simulink model "big2"  (R2023b)
settings: Solver=VariableStepAuto  StartTime=0.0  StopTime=500  RelTol=1e-3
libraries: simulink x2, aerolibasang x2, simulink_extras x2, aerolibanim x1
(part 3 of 3)

== matlab function big2/Subsystem/Subsystem3/MATLAB Function4 ==
  data: alpha input; DNDR output; beta input
% function DNDR = ddo_lookup(alpha, beta)
%     % Initialize output
%     DNDR = 0; % Ensure DLDN is scalar and fixed size
% 
%     % Declare persistent variables to hold constant data
%     persistent alpha_values beta_values data num_alpha num_beta
% 
%     if isempty(alpha_values)
%         % Initialize alpha and beta values in the table
%         alpha_values = [-10, -5, 0, 5, 10, 15, 20, 25, 30, 35, 40, 45];
%         beta_values  = [-30, -20, -10, 0, 10, 20, 30];
% 
%         num_alpha = length(alpha_values);
%         num_beta = length(beta_values);
% 
%         % Data matrix corresponding to beta (rows) and alpha (columns)
%          data = [
%         -.018, -.052, -.052, -.052, -.054, -.049, -.059, -.051, -.030, -.037, -.026, -.013; % Row for beta = -30
%         -.028, -.051, -.043, -.046, -.045, -.049, -.057, -.052, -.030, -.033, -.030, -.008; % Row for beta = -20°
%         -.037, -.041, -.038, -.040, -.040, -.038, -.037, -.030, -.027, -.024, -.019, -.013; % Row for beta = -10°
%         -.048, -.045, -.045, -.045, -.044, -.045, -.047, -.048, -.049, -.045, -.033, -.016; % Row for beta = 0°
%         -.043, -.044, -.041, -.041, -.040, -.038, -.034, -.035, -.035, -.029, -.022, -.009; % Row for beta = 10°
%         -.052, -.034, -.036, -.036, -.035, -.028, -.024, -.023, -.020, -.016, -.010, -.014; % Row for beta = 20°
%         -.062, -.034, -.027, -.028, -.027, -.027, -.023, -.023, -.019, -.009, -.025, -.010; % Row for beta = 30°
%     ];
%     end
% 
%     % Ensure alpha is within the range; if not, use the closest value
%     alpha_index = int32(1);
%     min_alpha_diff = abs(alpha - alpha_values(1));
%     for i = int32(2):int32(num_alpha)
%         current_diff = abs(alpha - alpha_values(i));
%         if current_diff < min_alpha_diff
%             min_alpha_diff = current_diff;
%             alpha_index = i;
%         end
%     end
% 
%     % Ensure beta is within the range; if not, use the closest value
%     beta_index = int32(1);
%     min_beta_diff = abs(beta - beta_values(1));
%     for i = int32(2):int32(num_beta)
%         current_diff = abs(beta - beta_values(i));
%         if current_diff < min_beta_diff
%             min_beta_diff = current_diff;
%             beta_index = i;
%         end
%     end
% 
%     % Retrieve the corresponding value from the data table
%     DNDR = data(beta_index, alpha_index);
% end
% 
function DNDR = ddo_lookup(alpha, beta)
    % Initialize output
    DNDR = 0; % Ensure DNDR is scalar and fixed size

    % Declare persistent variables to hold constant data
    persistent alpha_values beta_values data num_alpha num_beta

    if isempty(alpha_values)
        % Initialize alpha and beta values in the table
        alpha_values = [-10, -5, 0, 5, 10, 15, 20, 25, 30, 35, 40, 45];
        beta_values  = [-30, -20, -10, 0, 10, 20, 30];

        num_alpha = length(alpha_values);
        num_beta = length(beta_values);

        % Data matrix corresponding to beta (rows) and alpha (columns)
        data = [
            -0.018, -0.052, -0.052, -0.052, -0.054, -0.049, -0.059, -0.051, -0.030, -0.037, -0.026, -0.013; % Beta = -30°
            -0.028, -0.051, -0.043, -0.046, -0.045, -0.049, -0.057, -0.052, -0.030, -0.033, -0.030, -0.008; % Beta = -20°
            -0.037, -0.041, -0.038, -0.040, -0.040, -0.038, -0.037, -0.030, -0.027, -0.024, -0.019, -0.013; % Beta = -10°
            -0.048, -0.045, -0.045, -0.045, -0.044, -0.045, -0.047, -0.048, -0.049, -0.045, -0.033, -0.016; % Beta = 0°
            -0.043, -0.044, -0.041, -0.041, -0.040, -0.038, -0.034, -0.035, -0.035, -0.029, -0.022, -0.009; % Beta = 10°
            -0.052, -0.034, -0.036, -0.036, -0.035, -0.028, -0.024, -0.023, -0.020, -0.016, -0.010, -0.014; % Beta = 20°
            -0.062, -0.034, -0.027, -0.028, -0.027, -0.027, -0.023, -0.023, -0.019, -0.009, -0.025, -0.010; % Beta = 30°
        ];
    end

    % Handle out-of-range alpha values
    if alpha <= alpha_values(1)
        alpha_lower = alpha_values(1);
        alpha_upper = alpha_values(1);
        alpha_idx_lower = int32(1);
        alpha_idx_upper = int32(1);
    elseif alpha >= alpha_values(num_alpha)
        alpha_lower = alpha_values(num_alpha);
        alpha_upper = alpha_values(num_alpha);
        alpha_idx_lower = int32(num_alpha);
        alpha_idx_upper = int32(num_alpha);
    else
        % Find indices for alpha
        alpha_idx_lower = int32(1);
        alpha_idx_upper = int32(1);
        for i = int32(1):(num_alpha - 1)
            if alpha_values(i) <= alpha && alpha < alpha_values(i+1)
                alpha_idx_lower = i;
                alpha_idx_upper = i + 1;
                break;
            end
        end
        alpha_lower = alpha_values(alpha_idx_lower);
        alpha_upper = alpha_values(alpha_idx_upper);
    end

    % Handle out-of-range beta values
    if beta <= beta_values(1)
        beta_lower = beta_values(1);
        beta_upper = beta_values(1);
        beta_idx_lower = int32(1);
        beta_idx_upper = int32(1);
    elseif beta >= beta_values(num_beta)
        beta_lower = beta_values(num_beta);
        beta_upper = beta_values(num_beta);
        beta_idx_lower = int32(num_beta);
        beta_idx_upper = int32(num_beta);
    else
        % Find indices for beta
        beta_idx_lower = int32(1);
        beta_idx_upper = int32(1);
        for i = int32(1):(num_beta - 1)
            if beta_values(i) <= beta && beta < beta_values(i+1)
                beta_idx_lower = i;
                beta_idx_upper = i + 1;
                break;
            end
        end
        beta_lower = beta_values(beta_idx_lower);
        beta_upper = beta_values(beta_idx_upper);
    end

    % Get the four surrounding data points for bilinear interpolation
    Q11 = data(beta_idx_lower, alpha_idx_lower);
    Q12 = data(beta_idx_lower, alpha_idx_upper);
    Q21 = data(beta_idx_upper, alpha_idx_lower);
    Q22 = data(beta_idx_upper, alpha_idx_upper);

    % Perform bilinear interpolation
    if (alpha_upper - alpha_lower) == 0 && (beta_upper - beta_lower) == 0
        % Point lies exactly on a data point
        DNDR = data(beta_idx_lower, alpha_idx_lower);
    elseif (alpha_upper - alpha_lower) == 0
        % Interpolate in beta direction only
        DNDR = Q11 + ((beta - beta_lower) / (beta_upper - beta_lower)) * (Q21 - Q11);
    elseif (beta_upper - beta_lower) == 0
        % Interpolate in alpha direction only
        DNDR = Q11 + ((alpha - alpha_lower) / (alpha_upper - alpha_lower)) * (Q12 - Q11);
    else
        % Full bilinear interpolation
        DNDR = (1 / ((alpha_upper - alpha_lower) * (beta_upper - beta_lower))) * ...
               (Q11 * (alpha_upper - alpha) * (beta_upper - beta) + ...
                Q21 * (alpha - alpha_lower) * (beta_upper - beta) + ...
                Q12 * (alpha_upper - alpha) * (beta - beta_lower) + ...
                Q22 * (alpha - alpha_lower) * (beta - beta_lower));
    end
end

== matlab function big2/Subsystem/Subsystem1/MATLAB Function2 ==
  data: alpha input; c_m output; el input
function c_m = compute_cm_fixed(alpha, el)
    % Embedded data
    data_CM_updated_data_full = [
        0.205, 0.168, 0.186, 0.196, 0.213, 0.251, 0.245, 0.238, 0.252, 0.231, 0.198, 0.192;
        0.081, 0.077, 0.107, 0.110, 0.110, 0.141, 0.127, 0.119, 0.133, 0.108, 0.081, 0.093;
        -0.046, -0.020, -0.009, -0.005, -0.006, 0.010, 0.006, -0.001, 0.014, 0.000, -0.013, 0.032;
        -0.174, -0.145, -0.121, -0.127, -0.129, -0.102, -0.097, -0.113, -0.087, -0.084, -0.069, -0.006;
        -0.259, -0.202, -0.184, -0.193, -0.199, -0.150, -0.160, -0.167, -0.104, -0.076, -0.041, -0.005
    ];

    % Map Alpha and EL into indices and interpolate
    scaled_alpha = 0.2 * alpha;
    k = floor(scaled_alpha);
    k = max(-2, min(k, 8)); % Constrain within bounds
    da = scaled_alpha - k;
    l = k + sign(1.1 * da);
    l = max(-1, min(l, 8)); % Constrain within bounds

    % Adjust indices for MATLAB (1-based indexing)
    k_index = k + 3;
    l_index = l + 3;

    scaled_el = el / 12.5;
    m = floor(scaled_el);
    m = max(-2, min(m, 2)); % Constrain within bounds
    de = scaled_el - m;
    n = m + sign(1.1 * de);
    n = max(-2, min(n, 2)); % Constrain within bounds

    % Adjust indices for MATLAB (1-based indexing)
    m_index = m + 3;
    n_index = n + 3;

    % Interpolate values
    t = data_CM_updated_data_full(m_index, k_index);
    u = data_CM_updated_data_full(n_index, k_index);
    v = t + abs(da) * (data_CM_updated_data_full(m_index, l_index) - t);
    w = u + abs(da) * (data_CM_updated_data_full(n_index, l_index) - u);

    % Final interpolation
    c_m = v + (w - v) * abs(de);
end

== matlab function big2/Subsystem/Subsystem1/MATLAB Function3 ==
  data: alpha input; c_l output; beta input
function c_l = compute_cl_fixed(alpha, beta)
    % Embedded data
    data_CL_updated_data_full = [
        -0.001, -0.004, -0.008, -0.012, -0.016, -0.019, -0.020, -0.020, -0.015, -0.008, -0.013, -0.015;
        -0.003, -0.009, -0.017, -0.024, -0.030, -0.034, -0.040, -0.037, -0.016, -0.002, -0.010, -0.019;
        -0.001, -0.010, -0.020, -0.030, -0.039, -0.044, -0.050, -0.049, -0.023, -0.006, -0.014, -0.027;
        0.000, -0.010, -0.022, -0.034, -0.047, -0.046, -0.059, -0.061, -0.033, -0.036, -0.035, -0.035;
        0.007, -0.010, -0.023, -0.034, -0.049, -0.046, -0.068, -0.071, -0.060, -0.058, -0.062, -0.059;
        0.009, -0.011, -0.023, -0.037, -0.050, -0.047, -0.074, -0.079, -0.091, -0.076, -0.077, -0.076
    ];

    % Scale and map alpha into indices
    scaled_alpha = 0.2 * alpha;
    k = floor(scaled_alpha);                  % Find lower index
    k = max(-2, min(k, 8));                   % Constrain within bounds
    da = scaled_alpha - k;                    % Fractional part for interpolation
    l = k + sign(1.1 * da);                   % Find upper index
    l = max(-2, min(l, 8));                   % Constrain within bounds

    % Adjust indices for MATLAB (1-based indexing)
    k_index = k + 3;                          % Shift index for 1-based indexing
    l_index = l + 3;                          % Shift index for 1-based indexing

    % Scale and map beta into indices
    scaled_beta = 0.2 * abs(beta);
    m = floor(scaled_beta);                   % Find lower index
    m = max(0, min(m, 5));                    % Constrain within bounds
    db = scaled_beta - m;                     % Fractional part for interpolation
    n = m + sign(1.1 * db);                   % Find upper index
    n = max(0, min(n, 5));                    % Constrain within bounds

    % Adjust indices for MATLAB (1-based indexing)
    m_index = m + 1;                          % Shift index for 1-based indexing
    n_index = n + 1;                          % Shift index for 1-based indexing

    % Interpolation in the alpha dimension
    t = data_CL_updated_data_full(m_index, k_index); % Lower beta, lower alpha
    u = data_CL_updated_data_full(n_index, k_index); % Upper beta, lower alpha
    v = t + abs(da) * (data_CL_updated_data_full(m_index, l_index) - t); % Lower beta, interpolated alpha
    w = u + abs(da) * (data_CL_updated_data_full(n_index, l_index) - u); % Upper beta, interpolated alpha

    % Interpolation in the beta dimension
    c_l = v + (w - v) * abs(db);              % Final interpolated value
end

== matlab function big2/Subsystem/Subsystem1/MATLAB Function4 ==
  data: alpha input; c_n output; beta input
function c_n = compute_cn_fixed(alpha, beta)
    % Embedded data
    data_CN_updated_data_full = [
        0.018, 0.019, 0.018, 0.019, 0.019, 0.018, 0.013, 0.007, 0.004, -0.014, -0.017, -0.033;
        0.038, 0.042, 0.042, 0.042, 0.043, 0.039, 0.030, 0.017, 0.004, -0.035, -0.047, -0.057;
        0.056, 0.057, 0.059, 0.058, 0.058, 0.053, 0.032, 0.012, 0.002, -0.046, -0.071, -0.073;
        0.064, 0.077, 0.076, 0.074, 0.073, 0.057, 0.029, 0.007, 0.012, -0.034, -0.065, -0.041;
        0.074, 0.086, 0.093, 0.089, 0.080, 0.062, 0.049, 0.022, 0.028, -0.012, -0.002, -0.013;
        0.079, 0.090, 0.106, 0.106, 0.096, 0.080, 0.068, 0.030, 0.064, 0.015, 0.011, -0.001
    ];

    % Scale and map alpha into indices
    scaled_alpha = 0.2 * alpha;
    k = floor(scaled_alpha);                  % Find lower index
    k = max(-2, min(k, 8));                   % Constrain within bounds
    da = scaled_alpha - k;                    % Fractional part for interpolation
    l = k + sign(1.1 * da);                   % Find upper index
    l = max(-2, min(l, 8));                   % Constrain within bounds

    % Adjust indices for MATLAB (1-based indexing)
    k_index = k + 3;                          % Shift index for 1-based indexing
    l_index = l + 3;                          % Shift index for 1-based indexing

    % Scale and map beta into indices
    scaled_beta = 0.2 * abs(beta);
    m = floor(scaled_beta);                   % Find lower index
    m = max(0, min(m, 5));                    % Constrain within bounds
    db = scaled_beta - m;                     % Fractional part for interpolation
    n = m + sign(1.1 * db);                   % Find upper index
    n = max(0, min(n, 5));                    % Constrain within bounds

    % Adjust indices for MATLAB (1-based indexing)
    m_index = m + 1;                          % Shift index for 1-based indexing
    n_index = n + 1;                          % Shift index for 1-based indexing

    % Interpolation in the alpha dimension
    t = data_CN_updated_data_full(m_index, k_index); % Lower beta, lower alpha
    u = data_CN_updated_data_full(n_index, k_index); % Upper beta, lower alpha
    v = t + abs(da) * (data_CN_updated_data_full(m_index, l_index) - t); % Lower beta, interpolated alpha
    w = u + abs(da) * (data_CN_updated_data_full(n_index, l_index) - u); % Upper beta, interpolated alpha

    % Interpolation in the beta dimension
    c_n = v + (w - v) * abs(db);              % Final interpolated value
end

== matlab function big2/Subsystem/Subsystem1/MATLAB Function5 ==
  data: Beta input; c_y output; AIL input; RDR input
function c_y = compute_C_Y(Beta, AIL, RDR)
    % Compute C_Y based on Beta, AIL, and RDR
    c_y = -0.02 * Beta + (0.021 / 21.5) * AIL + (0.086 / 30) * RDR;
end

== matlab function big2/Subsystem/Subsystem/MATLAB Function ==
  data: U input; V_t output; V input; W input; alpha output; beta output
function [V_t, alpha, beta] = fcn(U, V, W)
    % Calculate the total velocity V_t
    V_t = sqrt(U^2 + V^2 + W^2);
    
    % Calculate alpha (angle of attack)
    % alpha = atan(W / U);
    alpha = atan2(W,U);
    % alpha = 0.698;
    
    % Calculate beta (side slip angle)
    % beta = atan(V / V_t);
    beta = asin(V / V_t);

    
    % Return the values
    % No need for 'y = V_t, alpha, beta;' as we already specify output variables
end

== matlab function big2/Subsystem2/MATLAB Function ==
  data: U input; V_t output; V input; W input; alpha output; beta output
function [V_t, alpha, beta] = fcn(U, V, W)
    % Calculate the total velocity V_t
    V_t = sqrt(U^2 + V^2 + W^2);
    
    % Calculate alpha (angle of attack)
    alpha = atan2(W , U);
    % alpha = 0.698;
    
    % Calculate beta (side slip angle)
    beta = asin(V / V_t);
    % beta = atan(V / V_t);
    
    % Return the values
    % No need for 'y = V_t, alpha, beta;' as we already specify output variables
end

== matlab function big2/Subsystem1/Subsystem/MATLAB Function ==
  data: L input; P_dot output; N input; I input; P input; Q input; R input
function P_dot = fcn(L,N,I,P,Q,R)
    % Extract inertia components from the 3x3 inertia matrix
    Ixx = I(1,1);
    Iyy = I(2,2);
    Izz = I(3,3);
    Ixz = I(1,3); % Assuming symmetric matrix
    
    % Compute Gamma
    Gamma = Ixx * Izz - Ixz^2;

    % Compute P_dot
    P_dot = (Izz * L + Ixz * N - (Izz * (Izz - Iyy) + Ixz^2) * Q * R ...
             + Ixz * (Ixx - Iyy + Izz) * P * Q) / Gamma;
    % P_dot = (Izz * L )/ Gamma;
